simulink model "mR52_MultiCPURecv"  (R2024a)
settings: Solver=FixedStepAuto  StartTime=0.0  StopTime=10.0  RelTol=1e-3  EnableMultiTasking=on
PreLoadFcn:
  | % NXP_MBDT_S32ZE callback: DO NOT REMOVE
  | mbd_s32ze.common.nxp.model_callbacks.preLoadFcn();
PostLoadFcn:
  | % NXP_MBDT_S32ZE callback: DO NOT REMOVE
  | mbd_s32ze.common.nxp.model_callbacks.postLoadFcn();
InitFcn:
  | % NXP_MBDT_S32ZE callback: DO NOT REMOVE
  | mbd_s32ze.common.nxp.model_callbacks.initFcn();
libraries: mbd_s32ze_cdd_library x5, mbd_s32ze_io_library x3
settings Model: DataDictionary=mR52_MultiCPURecv.sldd  Creator=scaliska  LastModifiedBy=nxf63265
settings SolverCC: AlgebraicLoopSolver=TrustRegion
settings DataIOCC: LimitDataPoints=on  SaveFormat=Array  ReturnWorkspaceOutputs=off
settings OptimizationCC: EnhancedBackFolding=on  PassReuseOutputArgsAs=Individual arguments  ZeroExternalMemoryAtStartup=off  ZeroInternalMemoryAtStartup=off  MaxStackSize=64  OptimizeBlockOrder=speed  DifferentSizesBufferReuse=on  OptimizationCustomize=off  EfficientTunableParamExpr=on
settings DebuggingCC: SolverPrmCheckMsg=warning  InheritedTsInSrcMsg=none  ParameterTunabilityLossMsg=error  UnconnectedInputMsg=warning  UnconnectedOutputMsg=warning  UnconnectedLineMsg=warning  AllowSymbolicDim=off  SFUnexpectedBacktrackingDiag=warning  SFNoUnconditionalDefaultTransitionDiag=warning  SFExecutionAtInitializationDiag=none  ArithmeticOperatorsInVariantConditions=warning
settings HardwareCC: ProdBitPerPointer=32  ProdBitPerSizeT=32  ProdBitPerPtrDiffT=32  ProdLargestAtomicInteger=Long  ProdLargestAtomicFloat=Double  ProdWordSize=32  ProdHWDeviceType=ARM Compatible->ARM Cortex
settings ModelReferenceCC: EnableRefExpFcnMdlSchedulingChecks=on  ModelReferenceNumInstancesAllowed=Single  PropagateSignalLabelsOutOfModel=off
settings SFSimCC: SimUseLocalCustomCode=off  MATLABDynamicMemAlloc=off  CustomCodeUndefinedFunction=UseInterfaceOnly
settings RTWCC: Description=Embedded Coder  SystemTargetFile=ert.tlc  HardwareBoard=NXP S32ZE2xx  TemplateMakefile=ert_default_tmf  RTWUseLocalCustomCode=off  Toolchain=NXP S32 Design Studio GCC (S32ZE)  GPUComputeCapability=3.5
settings CodeAppCC: ForceParamTrailComments=on  IgnoreCustomStorageClasses=off  MaxIdLength=63  OperatorAnnotations=on  SimulinkDataObjDesc=on  SFDataObjDesc=on  InsertBlockDesc=on
settings ERTTargetCC: SupportContinuousTime=on  ERTSrcFileBannerTemplate=mbd_s32ze_ert_code_template.cgt  ERTHdrFileBannerTemplate=mbd_s32ze_ert_code_template.cgt  ERTDataSrcFileTemplate=mbd_s32ze_ert_code_template.cgt  ERTDataHdrFileTemplate=mbd_s32ze_ert_code_template.cgt
settings ConfigComp: CovMetricSettings=dw  CovSaveCumulativeToWorkspaceVar=on  CovSaveSingleToWorkspaceVar=on  CovExternalEMLEnable=off  CovSFcnEnable=off

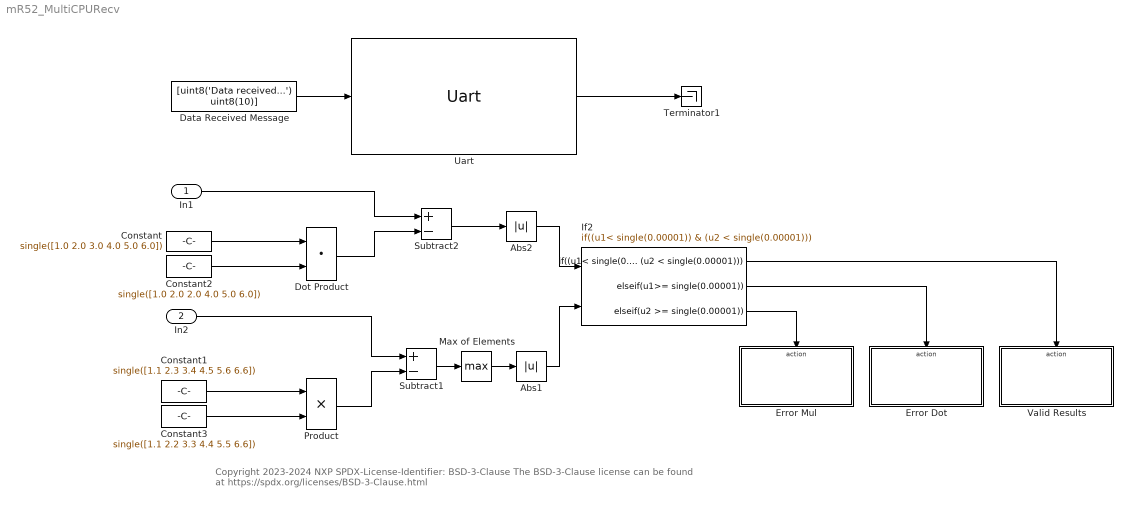
== system mR52_MultiCPURecv ==
  note: Copyright 2023-2024 NXP
      |
      | SPDX-License-Identifier: BSD-3-Clause
      | The BSD-3-Clause license can be found at https://spdx.org/licenses/BSD-3-Clause.html
  In1 : Inport  OutDataTypeStr=single
  In2 : Inport  Port=2  OutDataTypeStr=single  PortDimensions=[1 6]
  Abs1 : Abs  SaturateOnIntegerOverflow=off
  Abs2 : Abs  SaturateOnIntegerOverflow=off
  Constant : Constant  Value=single([1.0 2.0 3.0 4.0 5.0 6.0])  SampleTime=0
  Constant1 : Constant  Value=single([1.1 2.3 3.4 4.5 5.6 6.6])  SampleTime=0
  Constant2 : Constant  Value=single([1.0 2.0 2.0 4.0 5.0 6.0])  SampleTime=0
  Constant3 : Constant  Value=single([1.1 2.2 3.3 4.4 5.5 6.6])  SampleTime=0
  Data Received Message : Constant  Value=[uint8('Data received...') uint8(10)]  OutDataTypeStr=uint8
  Dot Product : DotProduct  OutDataTypeStr=single
  Error Dot : Subsystem  TreatAsAtomicUnit=on
  Error Mul : Subsystem  TreatAsAtomicUnit=on
  If2 : If  NumInputs=2  IfExpression=(u1< single(0.00001)) & (u2 < single(0.00001))  ElseIfExpressions=u1>= single(0.00001), u2 >= single(0.00001)  ShowElse=off
  Max of Elements : MinMax  Function=max
  Product : Product  OutDataTypeStr=single
  Subtract1 : Sum  Inputs=+-
  Subtract2 : Sum  Inputs=+-
  Terminator1 : Terminator
  Uart : mbd_s32ze_cdd_library/Uart  Priority=1  api_func=Uart_SyncSend  channel=UartChannel_0  baudrate=UART_BAUDRATE_1200  transfer_type=UART_SEND  timeout=1000000  text=<binary blob, 2545 chars, not shown>
  Valid Results : Subsystem  TreatAsAtomicUnit=on
  wires:
  In1/1 -> Subtract2/1
  Uart/1 -> Terminator1/1
  Data Received Message/1 -> Uart/1
  Dot Product/1 -> Subtract2/2
  In2/1 -> Subtract1/1
  Product/1 -> Subtract1/2
  Subtract1/1 -> Max of Elements/1
  Max of Elements/1 -> Abs1/1
  Abs1/1 -> If2/2
  Subtract2/1 -> Abs2/1
  Constant/1 -> Dot Product/1
  Constant2/1 -> Dot Product/2
  Constant1/1 -> Product/1
  Constant3/1 -> Product/2
  If2/1 -> Valid Results/Action
  If2/2 -> Error Dot/Action
  If2/3 -> Error Mul/Action
  Abs2/1 -> If2/1

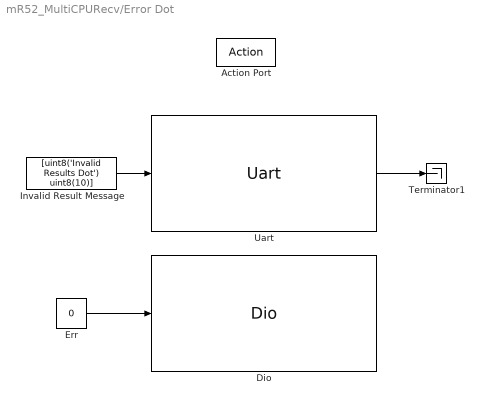
== system mR52_MultiCPURecv/Error Dot ==
  Action Port : ActionPort  ActionPortLabel=elseif(u1>= single(0.00001))
  Dio : mbd_s32ze_io_library/Dio  api_func=Dio_WriteChannel  channel=RED_D12_LED  channel_group=No channel groups configured  port=DioPort_0  gpioSim=off  text=<binary blob, 1229 chars, not shown>
  Err : Constant  Value=0  OutDataTypeStr=uint8
  Invalid Result Message : Constant  Value=[uint8('Invalid Results Dot') uint8(10)]  OutDataTypeStr=uint8
  Terminator1 : Terminator
  Uart : mbd_s32ze_cdd_library/Uart  api_func=Uart_SyncSend  channel=UartChannel_0  baudrate=UART_BAUDRATE_1200  transfer_type=UART_SEND  timeout=1000000  text=<binary blob, 2545 chars, not shown>
  wires:
  Invalid Result Message/1 -> Uart/1
  Uart/1 -> Terminator1/1
  Err/1 -> Dio/1

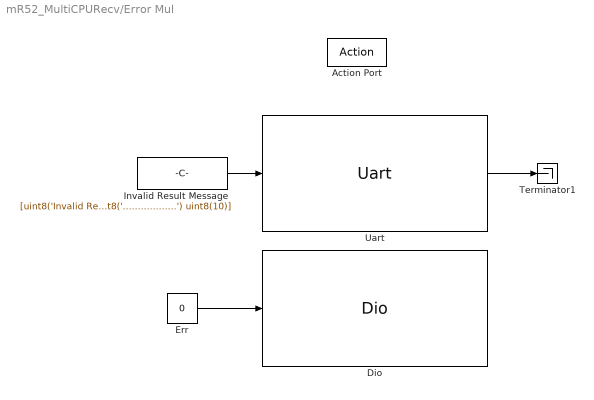
== system mR52_MultiCPURecv/Error Mul ==
  Action Port : ActionPort  ActionPortLabel=elseif( u2 >= single(0.00001))
  Dio : mbd_s32ze_io_library/Dio  api_func=Dio_WriteChannel  channel=RED_D12_LED  channel_group=No channel groups configured  port=DioPort_0  gpioSim=off  text=<binary blob, 1229 chars, not shown>
  Err : Constant  Value=0  OutDataTypeStr=uint8
  Invalid Result Message : Constant  Value=[uint8('Invalid Results Multiply') uint8(10) uint8('..................') uint8(10)]  OutDataTypeStr=uint8
  Terminator1 : Terminator
  Uart : mbd_s32ze_cdd_library/Uart  api_func=Uart_SyncSend  channel=UartChannel_0  baudrate=UART_BAUDRATE_1200  transfer_type=UART_SEND  timeout=1000000  text=<binary blob, 2545 chars, not shown>
  wires:
  Uart/1 -> Terminator1/1
  Invalid Result Message/1 -> Uart/1
  Err/1 -> Dio/1

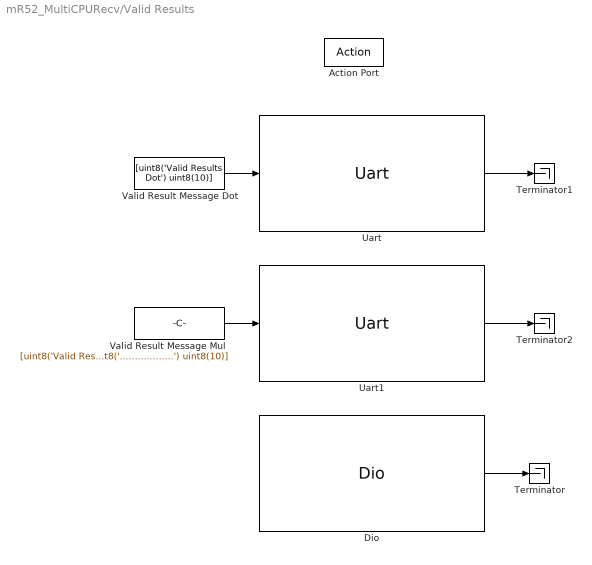
== system mR52_MultiCPURecv/Valid Results ==
  Action Port : ActionPort  ActionPortLabel=if((u1< single(0.00001)) & (u2 < single(0.00001)))
  Dio : mbd_s32ze_io_library/Dio  api_func=Dio_FlipChannel  channel=RED_D12_LED  channel_group=No channel groups configured  port=DioPort_0  gpioSim=off  text=<binary blob, 1229 chars, not shown>
  Terminator : Terminator
  Terminator1 : Terminator
  Terminator2 : Terminator
  Uart : mbd_s32ze_cdd_library/Uart  api_func=Uart_SyncSend  channel=UartChannel_0  baudrate=UART_BAUDRATE_1200  transfer_type=UART_SEND  timeout=1000000  text=<binary blob, 2545 chars, not shown>
  Uart1 : mbd_s32ze_cdd_library/Uart  api_func=Uart_SyncSend  channel=UartChannel_0  baudrate=UART_BAUDRATE_1200  transfer_type=UART_SEND  timeout=1000000  text=<binary blob, 2545 chars, not shown>
  Valid Result Message Dot : Constant  Value=[uint8('Valid Results Dot') uint8(10)]  OutDataTypeStr=uint8
  Valid Result Message Mul : Constant  Value=[uint8('Valid Results Multiply') uint8(10) uint8('..................') uint8(10)]  OutDataTypeStr=uint8
  wires:
  Valid Result Message Dot/1 -> Uart/1
  Uart/1 -> Terminator1/1
  Valid Result Message Mul/1 -> Uart1/1
  Uart1/1 -> Terminator2/1
  Dio/1 -> Terminator/1
